simulink model "modello_completo_simulink2019"  (R2019b)
settings: Solver=VariableStepAuto  StartTime=0.0  StopTime=10  RelTol=1e-3
values from neighbouring files (symbols this model uses):
  a = 0.35    [data.m]    (also in geodetic2nedS.m = 6378137)
  a1 = rho * D^4 * alpha1    (= 0.000388302366464)    [data.m]
  a2 = -rho * D^3 * alpha2 * (1 - omega)    (= 0.0037030698432)    [data.m]
  AHRS_bias = [0 0 0]    [data.m]
  AHRS_sample_time = 1/50    (= 0.02)    [data.m]
  AHRS_var = ([1 1 2] * pi/180).^2    [data.m]
  alpha1 = 0.0113    [data.m]
  alpha2 = -0.0091    [data.m]
  c = son2(1)    [Sonar_id.m]    (also in data.m = 0.19)
  current = [seaCurrent; 0; 0; 0]    [data.m]
  D = 0.076    [data.m]
  dead_zone_limit = 31.5    [data.m]
  DVL_sample_t = 1/12    (= 0.0833333333333)    [data.m]
  DVL_var1 = 0.005^2    (= 2.5e-05)    [data.m]
  DVL_var2 = 0.015^2    (= 0.000225)    [data.m]
  DVL_var3 = 0.023^2    (= 0.000529)    [data.m]
  gps_sample_t = 1    [data.m]
  H = eye(3)    [data.m]    (also in navigation_data.m)
  IMU_sample_time = 1/100    (= 0.01)    [data.m]
  initial = []    [data.m]
  INSP = unicode2native(inspectionDirection)    [data.m]
  Ki_bodypos1 = 0    [parametri_PID.m]
  Ki_bodypos2 = 0    [parametri_PID.m]
  Ki_bodypos3 = 0    [parametri_PID.m]
  Ki_bodypos4 = 0    [parametri_PID.m]
  Ki_bodypos5 = 0    [parametri_PID.m]
  Ki_depth1 = 0    [parametri_PID.m]
  Ki_depth2 = 0    [parametri_PID.m]
  Ki_depth3 = 0    [parametri_PID.m]
  Ki_depth4 = 0    [parametri_PID.m]
  Ki_depth5 = 0    [parametri_PID.m]
  Ki_latvel1 = 0    [parametri_PID.m]
  Ki_latvel2 = 0    [parametri_PID.m]
  Ki_latvel3 = 0    [parametri_PID.m]
  Ki_latvel4 = 0    [parametri_PID.m]
  Ki_latvel5 = 0    [parametri_PID.m]
  Ki_P1 = 0    [parametri_PID.m]
  Ki_P2 = 0    [parametri_PID.m]
  Ki_P3 = 0    [parametri_PID.m]
  Ki_P4 = 0    [parametri_PID.m]
  Ki_P5 = 0    [parametri_PID.m]
  Ki_R1 = 0    [parametri_PID.m]
  Ki_R2 = 0    [parametri_PID.m]
  Ki_R3 = 0    [parametri_PID.m]
  Ki_R4 = 0    [parametri_PID.m]
  Ki_R5 = 0    [parametri_PID.m]
  Ki_rel_or1 = 0    [parametri_PID.m]
  Ki_rel_or2 = 0    [parametri_PID.m]
  Ki_rel_or3 = 0    [parametri_PID.m]
  Ki_rel_or4 = 0    [parametri_PID.m]
  Ki_rel_or5 = 0    [parametri_PID.m]
  Ki_reldist1 = 0    [parametri_PID.m]
  Ki_reldist2 = 0    [parametri_PID.m]
  Ki_reldist3 = 0    [parametri_PID.m]
  Ki_reldist4 = 0    [parametri_PID.m]
  Ki_reldist5 = 0    [parametri_PID.m]
  Ki_surge1 = 0    [parametri_PID.m]
  Ki_surge2 = 0    [parametri_PID.m]
  Ki_surge3 = 0    [parametri_PID.m]
  Ki_surge4 = 0    [parametri_PID.m]
  Ki_surge5 = 0    [parametri_PID.m]
  Ki_yaw1 = 0    [parametri_PID.m]
  Ki_yaw2 = 0    [parametri_PID.m]
  Ki_yaw3 = 0    [parametri_PID.m]
  Ki_yaw4 = 0    [parametri_PID.m]
  Ki_yaw5 = 0    [parametri_PID.m]
  Kp_bodypos1 = 0    [parametri_PID.m]
  Kp_bodypos2 = 2    [parametri_PID.m]
  Kp_bodypos3 = 2    [parametri_PID.m]
  Kp_bodypos4 = 2    [parametri_PID.m]
  Kp_bodypos5 = 2    [parametri_PID.m]
  Kp_depth1 = 0    [parametri_PID.m]
  Kp_depth2 = 2    [parametri_PID.m]
  Kp_depth3 = 2    [parametri_PID.m]
  Kp_depth4 = 2    [parametri_PID.m]
  Kp_depth5 = 2    [parametri_PID.m]
  Kp_latvel1 = 0    [parametri_PID.m]
  Kp_latvel2 = 2    [parametri_PID.m]
  Kp_latvel3 = 2    [parametri_PID.m]
  Kp_latvel4 = 2    [parametri_PID.m]
  Kp_latvel5 = 2    [parametri_PID.m]
  Kp_P1 = 0    [parametri_PID.m]
  Kp_P2 = 2    [parametri_PID.m]
  Kp_P3 = 2    [parametri_PID.m]
  Kp_P4 = 2    [parametri_PID.m]
  Kp_P5 = 2    [parametri_PID.m]
  Kp_R1 = 0    [parametri_PID.m]
  Kp_R2 = 2    [parametri_PID.m]
  Kp_R3 = 2    [parametri_PID.m]
  Kp_R4 = 2    [parametri_PID.m]
  Kp_R5 = 2    [parametri_PID.m]
  Kp_rel_or1 = 0    [parametri_PID.m]
  Kp_rel_or2 = 2    [parametri_PID.m]
  Kp_rel_or3 = 2    [parametri_PID.m]
  Kp_rel_or4 = 2    [parametri_PID.m]
  Kp_rel_or5 = 2    [parametri_PID.m]
  Kp_reldist1 = 0    [parametri_PID.m]
  Kp_reldist2 = 2    [parametri_PID.m]
  Kp_reldist3 = 2    [parametri_PID.m]
  Kp_reldist4 = 2    [parametri_PID.m]
  Kp_reldist5 = 2    [parametri_PID.m]
  Kp_surge1 = 0    [parametri_PID.m]
  Kp_surge2 = 2    [parametri_PID.m]
  Kp_surge3 = 2    [parametri_PID.m]
  Kp_surge4 = 2    [parametri_PID.m]
  Kp_surge5 = 2    [parametri_PID.m]
  Kp_yaw1 = 0.6*6    (= 3.6)    [parametri_PID.m]
  Kp_yaw2 = 2    [parametri_PID.m]
  Kp_yaw3 = 2    [parametri_PID.m]
  Kp_yaw4 = 2    [parametri_PID.m]
  Kp_yaw5 = 2    [parametri_PID.m]
  M = M_rb + M_a    [Masse.m]
  M_inv = inv(M)    [Masse.m]
  n_max = 340    [data.m]
  num_cycle = 5    [data.m]    (also in navigation_data.m)
  omega = 0.1    [data.m]
  plot_smpl = 0.1    [data.m]
  ps_sample_t = 0.02    [data.m]
  ps_var = (5000/3)^2    (= 2777777.77778)    [data.m]
  pylonCenter = [ 43.723046 ... (first row only)    [missionB.m]
  ... (+4 more)
undefined symbols (not defined in the file or in its folder): DiscIntNeverNeededParam, s_data
libraries: simulink x3
(part 1 of 6)
settings Model: Creator=andrea  LastModifiedBy=Fabio
settings DebuggingCC: ArithmeticOperatorsInVariantConditions=warning
settings SFSimCC: CustomCodeUndefinedFunction=UseInterfaceOnly

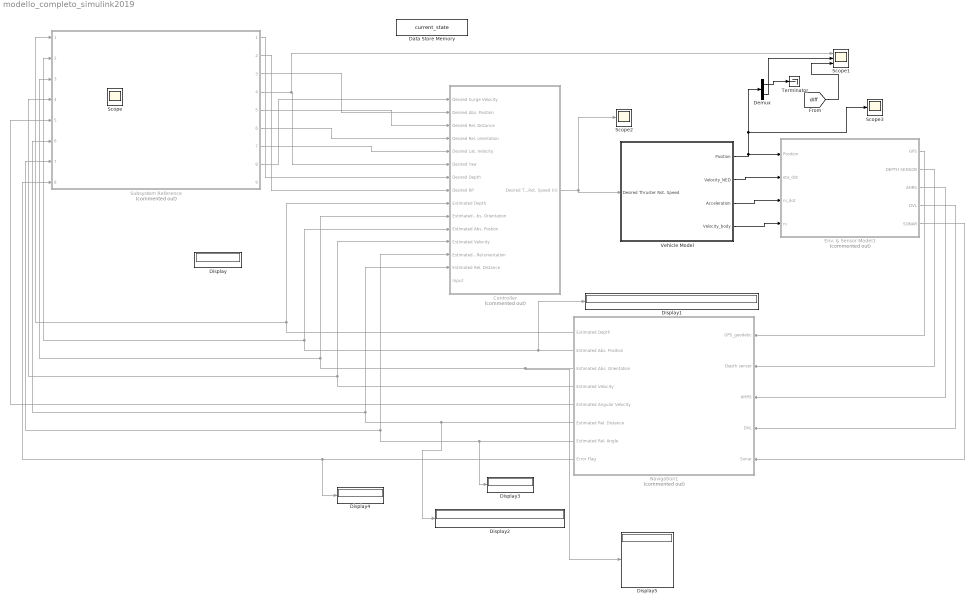
== system modello_completo_simulink2019 ==
  Controller : Subsystem  Commented=on
  Data Store Memory : DataStoreMemory  DataStoreName=current_state  ReadBeforeWriteMsg=warning  WriteAfterWriteMsg=warning  WriteAfterReadMsg=warning  ShowAdditionalParam=off
  Demux : Demux  Outputs=[5 1]
  Display{,1..5} (6 alike) : Display
  Env. & Sensor Model1 : Subsystem  Commented=on
  Navigation1 : Subsystem  Commented=on
  Scope1 : Scope  NumInputPorts=3
  Scope2 : Scope
  Scope3 : Scope
  Subsystem Reference : Subsystem  Commented=on  ReferencedSubsystem=mission_supervisor_sys
  Terminator : Terminator
  Vehicle Model : Subsystem
  Scope : Scope
  wires:
  Controller/1(Desired Thruster Rot. Speed (n)) -> Scope2/1, Vehicle Model/1(Desired Thruster Rot. Speed)
  Vehicle Model/1(Position) -> Env. & Sensor Model1/1(Position), Scope3/1, Demux/1
  Env. & Sensor Model1/2(DEPTH SENSOR) -> Navigation1/2(Depth sensor)
  Env. & Sensor Model1/3(AHRS) -> Navigation1/3(AHRS)
  Navigation1/1(Estimated Depth) -> Controller/9(Estimated Depth), Subsystem Reference/1
  Navigation1/2(Estimated Abs. Position) -> Display1/1, Controller/11(Estimated Abs. Postion), Subsystem Reference/2
  Navigation1/3(Estimated Abs. Orientation) -> Display5/1, Controller/10(Estimated Abs. Orientation), Subsystem Reference/3
  Navigation1/4(Estimated Velocity) -> Controller/12(Estimated Velocity), Subsystem Reference/4
  Vehicle Model/4(Velocity_body) -> Env. & Sensor Model1/4(ni)
  Navigation1/5(Estimated Angular Velocity) -> Subsystem Reference/5
  Navigation1/6(Estimated Rel. Distance) -> Display2/1, Controller/14(Estimated Rel. Distance), Subsystem Reference/6
  Navigation1/7(Estimated Rel. Angle) -> Display3/1, Controller/13(Estimated Rel.orientation), Subsystem Reference/7
  Navigation1/8(Error Flag) -> Display4/1, Subsystem Reference/8
  Vehicle Model/2(Velocity_NED) -> Env. & Sensor Model1/2(eta_dot)
  Vehicle Model/3(Acceleration) -> Env. & Sensor Model1/3(ni_dot)
  Env. & Sensor Model1/1(GPS) -> Navigation1/1(GPS_geodetic)
  Env. & Sensor Model1/4("DVL ") -> Navigation1/4(DVL)
  Env. & Sensor Model1/5(SONAR) -> Navigation1/5(Sonar)
  Subsystem Reference/8 -> Controller/1(Desired Surge Velocity)
  Subsystem Reference/7 -> Controller/5(Desired Lat. Velocity)
  Subsystem Reference/6 -> Controller/4(Desired Rel. orientation)
  Subsystem Reference/5 -> Controller/3(Desired Rel. Distance)
  Subsystem Reference/4 -> Scope1/1, Controller/6(Desired Yaw)
  Subsystem Reference/3 -> Controller/2(Desired Abs. Position)
  Subsystem Reference/2 -> Controller/8(Desired RP)
  Subsystem Reference/1 -> Controller/7(Desired Depth)
  ? -> Display/1, Controller/15(Input)
  Demux/1 -> Terminator/1
  Demux/2 -> Scope1/2
  [diff] -> Scope1/3

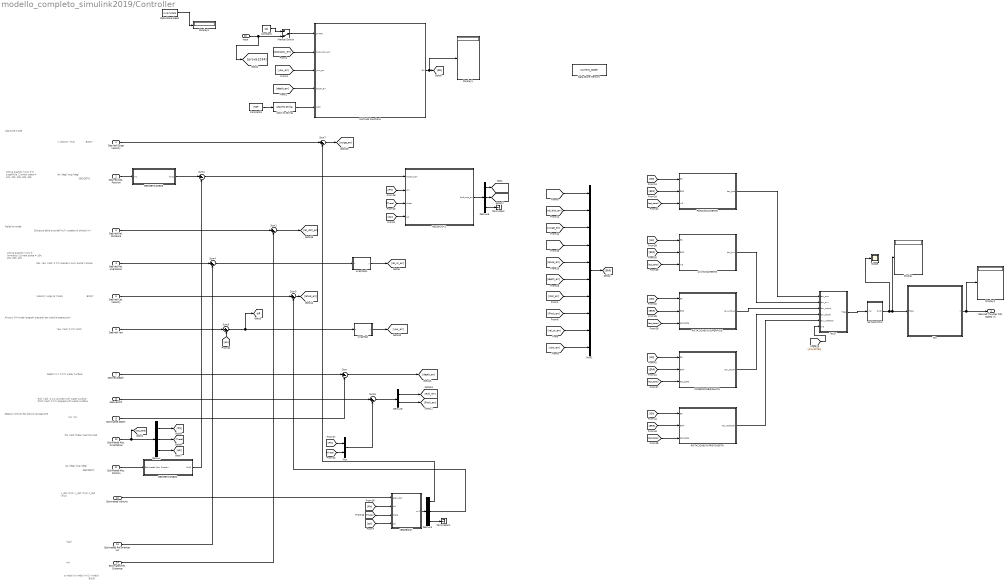
== system modello_completo_simulink2019/Controller ==
  note: lat (deg)
      | long (deg)
  note: (m)
  note: BODY
  note: x velocity (m/s)
  note: lat (deg)
      | long (deg)
  note: BODY
  note: p (rad/s)
      | q (rad/s)    mi2
      | r  (rad/s)
  note: GEODETIC
  note: BODY
  note: Relative mode
  note: Absolute mode
  note: GEODETIC
  note: Always ON mode (segnali presenti per tutte le operazioni)
  note: Roll (rad): 0 == aligned with water surface
      | Pitch (rad): 0 == aligned with water surface
  note: Velocity lungo la Y body
  note: Distanza della prua dell'AUV rispetto al pilone (m)
  note: Rel. Yaw (rad): 0 == quando il AUV punta il pilone
  note: Attiva quando il AUV è immerso.
      | Current state = 104, 201, 202, 401
  note: Attiva quando il AUV è in superficie.
      | Current state = 101, 102, 103, 402, 403
  note: Depth (m): 0 == water surface
  note: x_dot        (m/s)
      | y_dot          (m/s)
      | z_dot         (m/s)
  note: (rad)
  note: Segnali ricevuti dal blocco navigazione
  note: (m)
      | (m)
  note: Yaw (rad): 0 == north
  note: Phi (rad)
      | Theta (rad)
      | Psi(rad)
  Desired Surge Velocity : Inport
  Desired Abs. Position : Inport  Port=2  Unit=deg  PortDimensions=2
  Desired Rel. Distance : Inport  Port=3  Unit=m  PortDimensions=1
  Desired Rel. orientation : Inport  Port=4  Unit=rad  PortDimensions=1
  Desired Lat. Velocity : Inport  Port=5  Unit=m/s  PortDimensions=1
  Desired Yaw : Inport  Port=6  Unit=rad  PortDimensions=1
  Desired Depth : Inport  Port=7  Unit=m  PortDimensions=1
  Desired RP : Inport  Port=8  Unit=rad  PortDimensions=2
  Estimated Depth : Inport  Port=9  Unit=m  PortDimensions=1
  Estimated Abs. Orientation : Inport  Port=10  Unit=rad  PortDimensions=3
  Estimated Abs. Postion : Inport  Port=11  Unit=deg  PortDimensions=2
  Estimated Velocity : Inport  Port=12  Unit=m/s  PortDimensions=3
  Estimated Rel.orientation : Inport  Port=13  Unit=rad  PortDimensions=1
  Estimated Rel. Distance : Inport  Port=14  Unit=m  PortDimensions=1
  Input : Inport  Port=15
  ASCII to String : ASCIIToString
  AVVICINAMENTO : Subsystem
  Constant : Constant  Value=101
  Constant3 : Constant  Value=INSP  OutDataTypeStr=uint8
  Data Store Memory : DataStoreMemory  DataStoreName=current_state  ReadBeforeWriteMsg=warning  WriteAfterWriteMsg=warning  WriteAfterReadMsg=warning  ShowAdditionalParam=off
  Data Store Read : DataStoreRead  DataStoreName=current_state  SampleTime=0.1
  Demux : Demux  Outputs=3
  Demux1 : Demux  Outputs=3
  Demux5 : Demux  Outputs=3
  Demux6 : Demux  Outputs=2
  Display{,1..3} (4 alike) : Display
  GEODETIC2NED2 : Subsystem
  GEODETIC2NED3 : Subsystem
  IMMERSIONE/RISALITA : Subsystem
  MATLAB Function1 : MATLAB Function  TreatAsAtomicUnit=on  SystemSampleTime=0.1
  Manual Switch : ManualSwitch  CurrentSetting=0
  Mux : Mux  Inputs=2
  Mux1 : Mux  Inputs=10
  NED2BODY : MATLAB Function  TreatAsAtomicUnit=on
  NED2BODY1 : MATLAB Function  TreatAsAtomicUnit=on
  POSIZIONAMENTO : Subsystem
  ROTAZIONE IN PROFONDITA' : Subsystem
  ROTAZIONE IN SUPERFICIE : Subsystem
  SATURATION : Subsystem
  Scope : Scope
  Sum{,1..7} (8 alike) : Sum  Inputs=|+-
  T2n : Subsystem
  Tau2T : Subsystem
  Terminator : Terminator
  Terminator1 : Terminator
  wrapTopi : MATLAB Function  TreatAsAtomicUnit=on
  wrapTopi1 : MATLAB Function  TreatAsAtomicUnit=on
  Desired Thruster Rot. Speed (n) : Outport  Unit=rad/s  PortDimensions=7
  tag scope: diff=global
  wires:
  Estimated Abs. Orientation/1 -> [est_state], Demux/1
  Desired Depth/1 -> Sum/1
  Estimated Depth/1 -> Sum/2
  Mux/1 -> Sum6/2
  Desired RP/1 -> Sum6/1
  T2n/1(n) -> Desired Thruster Rot. Speed (n)/1, Display2/1
  Desired Lat. Velocity/1 -> Sum3/1
  Desired Rel. Distance/1 -> Sum1/1
  Estimated Rel. Distance/1 -> Sum1/2
  Sum2/1 -> NED2BODY1/1(abspos_err)
  Desired Abs. Position/1 -> GEODETIC2NED3/1(In1)
  GEODETIC2NED3/1(Out1) -> Sum2/1
  Estimated Abs. Postion/1 -> GEODETIC2NED2/1(Estimated Abs. Postion)
  GEODETIC2NED2/1(Out1) -> Sum2/2
  Demux1/1 -> Sum7/2
  Demux1/2 -> Sum3/2
  NED2BODY/1(mi1) -> Demux1/1
  Estimated Velocity/1 -> NED2BODY/1(eta1_dot)
  Estimated Rel.orientation/1 -> Sum4/2
  Demux/3 -> [psi]
  [psi] -> NED2BODY/4(psi)
  [psi] -> NED2BODY1/4(psi)
  Demux/2 -> [Theta]
  [Theta] -> Mux/2
  [Theta] -> NED2BODY1/3(theta)
  [Theta] -> NED2BODY/3(theta)
  Demux/1 -> [Phi]
  [Phi] -> Mux/1
  [Phi] -> NED2BODY/2(phi)
  [Phi] -> NED2BODY1/2(phi)
  Tau2T/1(Tdes) -> SATURATION/1(In2)
  SATURATION/1(Out2) -> Scope/1, Display/1, T2n/1(Tdes)
  Desired Rel. orientation/1 -> Sum4/1
  Desired Surge Velocity/1 -> Sum7/1
  [ERR] -> POSIZIONAMENTO/2(ERR)
  [EN] -> POSIZIONAMENTO/1(EN)
  Sum4/1 -> wrapTopi1/1(u)
  Desired Yaw/1 -> Sum5/1
  [psi] -> Sum5/2
  Sum/1 -> [depth_err]
  Sum3/1 -> [latvel_err]
  Sum1/1 -> [rel_dist_err]
  NED2BODY1/1(bodypos_err) -> Demux5/1
  Sum7/1 -> [surge_err]
  Demux5/1 -> [bodyposx_err]
  Demux5/2 -> [bodyposy_err]
  [EN] -> AVVICINAMENTO/1(EN)
  [ERR] -> AVVICINAMENTO/2(ERR)
  [ERR] -> ROTAZIONE IN SUPERFICIE/2(ERR)
  [ERR] -> IMMERSIONE/RISALITA/2(ERR)
  [EN] -> IMMERSIONE/RISALITA/1(EN)
  [ERR] -> ROTAZIONE IN PROFONDITA'/2(ERR)
  [EN] -> ROTAZIONE IN PROFONDITA'/1(EN)
  MATLAB Function1/1(EN) -> Display1/1, [EN]
  [bodyposx_err] -> Mux1/1
  [rel_dist_err] -> Mux1/2
  [surge_err] -> Mux1/3
  [bodyposy_err] -> Mux1/4
  [latvel_err] -> Mux1/5
  [depth_err] -> Mux1/6
  Mux1/1 -> [ERR]
  [Roll_err] -> Mux1/7
  [Pitch_err] -> Mux1/8
  [rel_or_err] -> Mux1/9
  [yaw_err] -> Mux1/10
  [EN] -> ROTAZIONE IN SUPERFICIE/1(EN)
  POSIZIONAMENTO/1(tau_pos) -> Tau2T/1(tau_pos)
  AVVICINAMENTO/1(tau_avv) -> Tau2T/2(tau_avv)
  ROTAZIONE IN SUPERFICIE/1(tau_rotsup) -> Tau2T/3(tau_rotsup)
  IMMERSIONE/RISALITA/1(tau_depth) -> Tau2T/4(tau_depth)
  ROTAZIONE IN PROFONDITA'/1(tau_rotdepth) -> Tau2T/5(tau_rotdepth)
  [depth_err] -> MATLAB Function1/4(depth_err)
  [yaw_err] -> MATLAB Function1/3(yaw_err)
  [bodyposx_err] -> MATLAB Function1/2(bodyposx_err)
  Constant/1 -> Manual Switch/1
  Data Store Read/1 -> Display3/1
  Manual Switch/1 -> MATLAB Function1/1(STATE)
  Demux5/3 -> Terminator/1
  wrapTopi1/1(y) -> [rel_or_err]
  wrapTopi/1(y) -> [yaw_err]
  Sum6/1 -> Demux6/1
  Demux6/1 -> [Roll_err]
  Demux6/2 -> [Pitch_err]
  ASCII to String/1 -> MATLAB Function1/5(INSP)
  Constant3/1 -> ASCII to String/1
  [est_state] -> POSIZIONAMENTO/3(In3)
  [est_state] -> AVVICINAMENTO/3(In3)
  [est_state] -> ROTAZIONE IN SUPERFICIE/3(est_state)
  [est_state] -> IMMERSIONE/RISALITA/3(est_state)
  [est_state] -> ROTAZIONE IN PROFONDITA'/3(est_state)
  Demux1/3 -> Terminator1/1
  Input/1 -> [prova1234], Manual Switch/2
  [prova1234] -> Tau2T/6(In6)
  Sum5/1 -> [diff], wrapTopi/1(u)
